simulink model "LiuWeihao_simulink"  (R2021a)
settings: Solver=FixedStepAuto  StartTime=0.0  StopTime=500  FixedStep=0.005  RelTol=1e-8
settings Model: Creator=l_w_h  LastModifiedBy=l_w_h

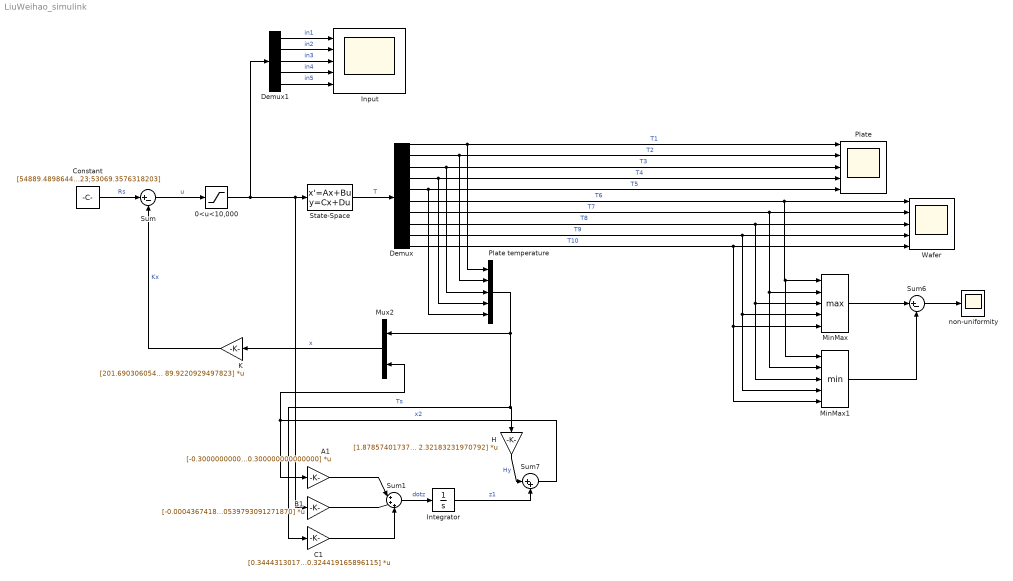
== system LiuWeihao_simulink ==
  0<u<10,000 : Saturate  UpperLimit=10e4  LowerLimit=0
  A1 : Gain  Gain=[-0.300000000000000 0 0 0 0;0 -0.300000000000000 -6.93889390390723e-18 0 0;0 6.93889390390723e-18 -0.300000000000000 0 0;0 0 0 -0.300000000000000 6.93889390390723e-18;0 0 0 -3.46944695195361e-18 -0.300000000000000]  Multiplication=Matrix(K*u)
  B1 : Gain  Gain=[-0.000436741821281746 -0.000201465857250265 0 0 0;-6.71552857500885e-05 -0.000426624199007793 -0.000144428193774131 0 0;0 -8.66569162644783e-05 -0.000419989912703969 -0.000131560849563564 0;0 0 -9.39720354025459e-05 -0.000418421215569420 -0.000125814427560046;0 0 0 -9.78556658800356e-05 -0.000539793091271870]  Multiplication=Matrix(K*u)
  C1 : Gain  Gain=[0.344431301747057 -0.0117512821095320 -0.0385532259236173 0 0;-0.00391709403651067 0.328438474570554 -0.00521863281406086 -0.0251759540060748 0;-0.00771064518472346 -0.00313117968843653 0.330223715802212 -0.00332379586198954 -0.0219313013531552;0 -0.0107896945740321 -0.00237413990142110 0.330533705208892 -0.0231878429325686;0 0 -0.0121840563073084 -0.0180054811749444 0.324419165896115]  Multiplication=Matrix(K*u)
  Constant : Constant  Value=[54889.4898644001;60552.2126497191;53779.9848506266;51528.7868501523;53069.3576318203]
  Demux : Demux  Outputs=10
  Demux1 : Demux  Outputs=5
  H : Gain  Gain=[1.87857401737166 0.866572666906799 0 0 0;0.288857555635600 1.83505470826210 0.621234420380753 0 0;0 0.372740652228452 1.80651840313430 0.565887628915702 0;0 0 0.404205449225502 1.79977090716645 0.541170327886501;0 0 0 0.420910255022834 2.32183231970792]  Multiplication=Matrix(K*u)
  Input : Scope  NumInputPorts=5
  Integrator : Integrator
  K : Gain  Gain=[201.690306054278 87.8583492911557 19.1672442465896 2.24733787981690 -0.216931739410048 113.494330532729 43.0115621820785 8.10286841568017 0.803578895911601 -0.110839651801959;87.8583492911553 196.200340440051 67.0638801209133 16.0626647370285 2.57703251064413 44.4644591138252 76.5731017337843 27.2230064504165 6.18088621949413 0.861726282607638;19.1672442465892 67.0638801209131 170.170457785174 59.3453918897096 18.1930491873680 8.30428287884535 27.9236385185415 63.7600949626428 24.0551774956149 6.99425512340878;2.24733787981663 16.0626647370288 59.3453918897098 168.158640161621 74.5830629095694 0.770794031150246 6.47736947465096 24.5156033611468 62.8815339723936 30.1389028390661;-0.216931739409030 2.57703251064509 18.1930491873683 74.5830629095689 234.037574264448 -0.129924886185211 0.942353448867821 7.24920108069418 30.5433964300734 89.9220929497823]  Multiplication=Matrix(K*u)
  MinMax : MinMax  Function=max  Inputs=5
  MinMax1 : MinMax  Inputs=5
  Mux2 : Mux  Inputs=2
  Plate : Scope  NumInputPorts=5
  Plate temperature : Mux  Inputs=5
  State-Space : StateSpace  A=[-0.117855659679215 0.0620590628252506 0 0 0 0.0557965968539647 0 0 0 0;0.0206863542750835 -0.120972267946796 0.0444893168177479 0 0 0 0.0557965968539647 0 0 0;0 0.0266935900906488 -0.123015877698588 0.0405256907539742 0 0 0 0.0557965968539647 0 0;0 0 0.0289469219671245 -0.123499095427663 0.0387555766065743 0 0 0 0.0557965968539647 0;0 0 0 0.0301432262495578 -0.0860418872487965 0 0 0 0 0.0557965968539647;0.140956950866225 0 0 0 0 -0.195181962892381 0.0483518057400637 0 0 0;0 0.140956950866225 0 0 0 0.0161172685800212 -0.197610192238130 0.0346627665057913 0 0;0 0 0.140956950866225 0 0 0 0.0207976599034748 -0.199202420951047 0.0315746038952554 0;0 0 0 0.140956950866225 0 0 0 0.0225532884966110 -0.199578908263339 0.0301954626144110;0 0 0 0 0.140956950866225 0 0 0 0.0234853598112085 -0.170449658094751]  B=[0.000232485820224853 0 0 0 0;0 0.000232485820224853 0 0 0;0 0 0.000232485820224853 0 0;0 0 0 0.000232485820224853 0;0 0 0 0 0.000232485820224853;0 0 0 0 0;0 0 0 0 0;0 0 0 0 0;0 0 0 0 0;0 0 0 0 0]  C=[1 0 0 0 0 0 0 0 0 0;0 1 0 0 0 0 0 0 0 0;0 0 1 0 0 0 0 0 0 0;0 0 0 1 0 0 0 0 0 0;0 0 0 0 1 0 0 0 0 0;0 0 0 0 0 1 0 0 0 0;0 0 0 0 0 0 1 0 0 0;0 0 0 0 0 0 0 1 0 0;0 0 0 0 0 0 0 0 1 0;0 0 0 0 0 0 0 0 0 1]  D=[0 0 0 0 0;0 0 0 0 0;0 0 0 0 0;0 0 0 0 0;0 0 0 0 0;0 0 0 0 0;0 0 0 0 0;0 0 0 0 0;0 0 0 0 0;0 0 0 0 0]  InitialCondition=[114.583333333333;114.583333333333;114.583333333333;114.583333333333;114.688014403292;25;25;25;25;25]  ParameterTunability=Unconstrained
  Sum : Sum  Inputs=|+-
  Sum1 : Sum  Inputs=|+++
  Sum6 : Sum  Inputs=|+-
  Sum7 : Sum  Inputs=|++
  Wafer : Scope  NumInputPorts=5
  non-uniformity : Scope
  wires:
  Demux/5 -> Plate temperature/5, Plate/5  "T5"
  Demux/9 -> Wafer/4, MinMax1/4, MinMax/4  "T9"
  Demux/3 -> Plate temperature/3, Plate/3  "T3"
  Demux/7 -> Wafer/2, MinMax1/2, MinMax/2  "T7"
  Demux/8 -> Wafer/3, MinMax1/3, MinMax/3  "T8"
  Demux/1 -> Plate temperature/1, Plate/1  "T1"
  Demux/2 -> Plate temperature/2, Plate/2  "T2"
  Demux/4 -> Plate temperature/4, Plate/4  "T4"
  Constant/1 -> Sum/1  "Rs"
  Plate temperature/1 -> H/1, C1/1, Mux2/1  "Ts"
  B1/1 -> Sum1/2
  C1/1 -> Sum1/3
  Sum1/1 -> Integrator/1  "dotz"
  Integrator/1 -> Sum7/2  "z1"
  K/1 -> Sum/2  "Kx"
  Mux2/1 -> K/1  "x"
  State-Space/1 -> Demux/1  "T"
  Demux/10 -> Wafer/5, MinMax1/5, MinMax/5  "T10"
  Demux/6 -> MinMax1/1, MinMax/1, Wafer/1  "T6"
  MinMax/1 -> Sum6/1
  MinMax1/1 -> Sum6/2
  Sum6/1 -> non-uniformity/1
  Demux1/1 -> Input/1  "in1"
  Demux1/2 -> Input/2  "in2"
  Demux1/3 -> Input/3  "in3"
  Demux1/4 -> Input/4  "in4"
  Demux1/5 -> Input/5  "in5"
  H/1 -> Sum7/1  "Hy"
  Sum7/1 -> A1/1, Mux2/2  "x2"
  Sum/1 -> 0<u<10,000/1  "u"
  0<u<10,000/1 -> Demux1/1, B1/1, State-Space/1
  A1/1 -> Sum1/1
